simulink model "simRobotArmWith2Links"  (R2014b)
settings: Solver=ode5  StartTime=0.0  StopTime=tf  FixedStep=dt  MaxStep=dtmax  RelTol=1e-3
values from neighbouring files (symbols this model uses):
  alpha = 1    [robotArmWith2Links.m]    (also in threeLinkFTC.m; twoLinkFTC.m; twoLinkFTCwAdaptive.m)
  Ar = [0 5; -30 -30]    [robotArmWith2Links.m]    (also in threeLinkFTC.m = [0 1; -5 -5]; twoLinkFTC.m = [0 10; -40 -40]; twoLinkFTCwAdaptive.m = [0 5; -250 -250])
  Arm1 = [0 1; -wn^2 -2*ksi*wn]    [robotArmWith2Links.m]    (also in threeLinkFTC.m; twoLinkFTC.m; twoLinkFTCwAdaptive.m)
  Bfault = [0 0; 0 1]    [robotArmWith2Links.m]    (also in threeLinkFTC.m; twoLinkFTC.m; twoLinkFTCwAdaptive.m)
  Brm1 = [0 wn^2]'    [robotArmWith2Links.m]    (also in threeLinkFTC.m; twoLinkFTC.m; twoLinkFTCwAdaptive.m)
  dt = 1e-3    (= 0.001)    [robotArmWith2Links.m]
  dtFC = dt    (= 0.001)    [robotArmWith2Links.m]
  epsilon = 0.5    [robotArmWith2Links.m]    (also in threeLinkFTC.m; twoLinkFTC.m; twoLinkFTCwAdaptive.m)
  g = 9.81    [robotArmWith2Links.m]    (also in threeLinkFTC.m; twoLinkFDIbasisComparison.m; twoLinkFTC.m; twoLinkFTCwAdaptive.m)
  I1 = 8.33e-2    (= 0.0833)    [robotArmWith2Links.m]    (also in threeLinkFTC.m = 0.0833333333333; twoLinkFDIbasisComparison.m = 0.0833333333333; twoLinkFTC.m = 0.0833333333333; twoLinkFTCwAdaptive.m = 0.0833333333333)
  I2 = 8.33e-2    (= 0.0833)    [robotArmWith2Links.m]    (also in threeLinkFTC.m = 0.0833333333333; twoLinkFDIbasisComparison.m = 0.0833333333333; twoLinkFTC.m = 0.0833333333333; twoLinkFTCwAdaptive.m = 0.0833333333333)
  K1 = 2*wn*ksi    (= 87.9645943005)    [robotArmWith2Links.m]    (also in threeLinkFTC.m = 8.79645943005; twoLinkFTC.m; twoLinkFTCwAdaptive.m = 43.9822971503)
  K2 = wn^2    (= 986.960440109)    [robotArmWith2Links.m]    (also in threeLinkFTC.m = 39.4784176044; twoLinkFTC.m; twoLinkFTCwAdaptive.m)
  l1 = 1    [robotArmWith2Links.m]    (also in threeLinkFTC.m; twoLinkFDIbasisComparison.m; twoLinkFTC.m; twoLinkFTCwAdaptive.m)
  l2 = 1    [robotArmWith2Links.m]    (also in threeLinkFTC.m; twoLinkFDIbasisComparison.m; twoLinkFTC.m; twoLinkFTCwAdaptive.m)
  lc1 = l1/2    (= 0.5)    [robotArmWith2Links.m]    (also in threeLinkFTC.m; twoLinkFDIbasisComparison.m; twoLinkFTC.m; twoLinkFTCwAdaptive.m)
  lc2 = l2/2    (= 0.5)    [robotArmWith2Links.m]    (also in threeLinkFTC.m; twoLinkFDIbasisComparison.m; twoLinkFTC.m; twoLinkFTCwAdaptive.m)
  m1 = 1    [robotArmWith2Links.m]    (also in threeLinkFTC.m; twoLinkFDIbasisComparison.m; twoLinkFTC.m; twoLinkFTCwAdaptive.m)
  m2 = 1    [robotArmWith2Links.m]    (also in threeLinkFTC.m; twoLinkFDIbasisComparison.m; twoLinkFTC.m; twoLinkFTCwAdaptive.m)
  q0 = [80 20]'*pi/180    [robotArmWith2Links.m]    (also in threeLinkFTC.m = [90 0 0]'*pi/180; twoLinkFDIbasisComparison.m = [90 0]'*pi/180; twoLinkFTC.m = [90 0]'*pi/180; twoLinkFTCwAdaptive.m = [90 0]'*pi/180)
  qdot0 = [0 0]'    [robotArmWith2Links.m]    (also in threeLinkFTC.m = [0 0 0]'*pi/180; twoLinkFDIbasisComparison.m = [0 0]'*pi/180; twoLinkFTC.m = [0 0]'*pi/180; twoLinkFTCwAdaptive.m = [0 0]'*pi/180)
  r0 = [0 0]'    [robotArmWith2Links.m]    (also in threeLinkFTC.m; twoLinkFTC.m; twoLinkFTCwAdaptive.m)
  rmax = inf*[50*pi/180 inf]'    [robotArmWith2Links.m]    (also in threeLinkFTC.m; twoLinkFTC.m; twoLinkFTCwAdaptive.m)
  rmin = -rmax    [robotArmWith2Links.m]    (also in threeLinkFTC.m; twoLinkFTC.m; twoLinkFTCwAdaptive.m)
  visualFlag = 0    [robotArmWith2Links.m]    (also in twoLinkFDIbasisComparison.m; twoLinkFTC.m; twoLinkFTCwAdaptive.m)
  visualizationDataFlag = 1    [robotArmWith2Links.m]    (also in twoLinkFDIbasisComparison.m; twoLinkFTC.m; twoLinkFTCwAdaptive.m)
undefined symbols (not defined in the file or in its folder): twolinkplot
libraries: simulink x1
(part 1 of 2)
settings Model: Creator=alp.marangoz  LastModifiedBy=alpmarangoz
settings SolverCC: AutoInsertRateTranBlk=on
settings DataIOCC: SignalLoggingSaveFormat=ModelDataLogs
settings OptimizationCC: InlineParams=on  InlineInvariantSignals=on  ExpressionDepthLimit=2147483647  EfficientFloat2IntCast=on
settings DebuggingCC: UnderspecifiedInitializationDetection=Classic  MergeDetectMultiDrivingBlocksExec=none  FcnCallInpInsideContextMsg=UseLocalSettings  UniqueDataStoreMsg=error  StateNameClashWarn=warning
settings GRTTargetCC: CombineOutputUpdateFcns=off  GRTInterface=on

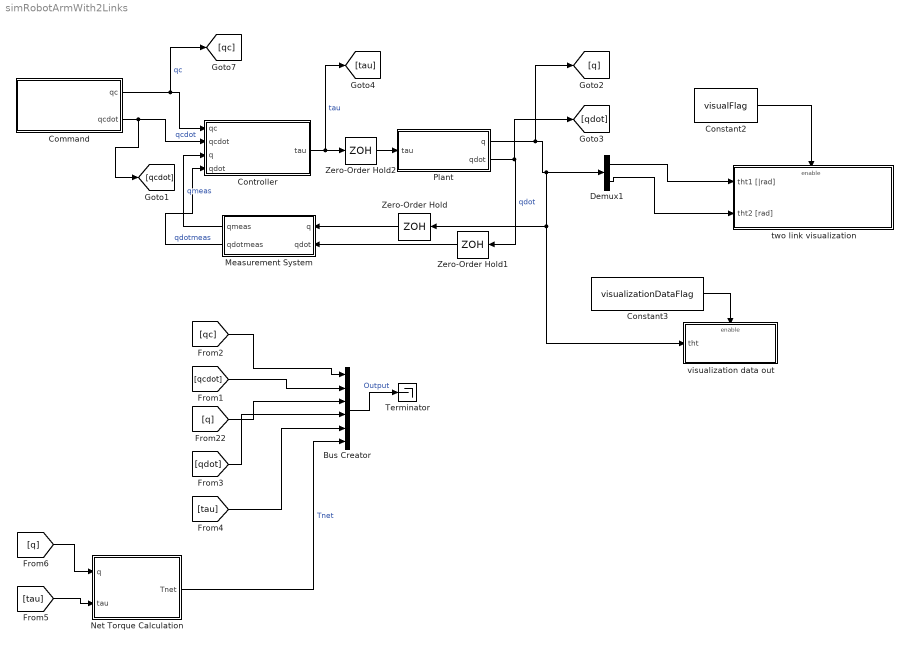
== system simRobotArmWith2Links ==
  Bus Creator : BusCreator  Inputs=6
  Command : Subsystem  TreatAsAtomicUnit=on  SystemSampleTime=dtFC
  Constant2 : Constant  Value=visualFlag
  Constant3 : Constant  Value=visualizationDataFlag
  Controller : Subsystem  TreatAsAtomicUnit=on  SystemSampleTime=dtFC
  Demux1 : Demux  Outputs=2
  Measurement System : Subsystem  TreatAsAtomicUnit=on  SystemSampleTime=dtFC
  Net Torque Calculation : Subsystem
  Plant : Subsystem  TreatAsAtomicUnit=on
  Terminator : Terminator
  Zero-Order Hold : ZeroOrderHold  SampleTime=dtFC
  Zero-Order Hold1 : ZeroOrderHold  SampleTime=dtFC
  Zero-Order Hold2 : ZeroOrderHold  SampleTime=dtFC
  two link visualization : Subsystem
  visualization data out : Subsystem  TreatAsAtomicUnit=on
  wires:
  Constant2/1 -> two link visualization/Enable
  Demux1/1 -> two link visualization/1(tht1 [|rad])
  Demux1/2 -> two link visualization/2(tht2 [rad])
  Command/1(qc) -> [qc], Controller/1(qc)  "qc"
  Command/2(qcdot) -> [qcdot], Controller/2(qcdot)  "qcdot"
  Measurement System/1(qmeas) -> Controller/3(q)  "qmeas"
  Measurement System/2(qdotmeas) -> Controller/4(qdot)  "qdotmeas"
  Constant3/1 -> visualization data out/Enable
  Controller/1(tau) -> [tau], Zero-Order Hold2/1  "tau"
  Plant/1(q) -> [q], Demux1/1, visualization data out/1(tht), Zero-Order Hold/1
  Plant/2(qdot) -> [qdot], Zero-Order Hold1/1  "qdot"
  Zero-Order Hold/1 -> Measurement System/1(q)
  Zero-Order Hold1/1 -> Measurement System/2(qdot)
  Zero-Order Hold2/1 -> Plant/1(tau)
  Bus Creator/1 -> Terminator/1  "Output"
  [qcdot] -> Bus Creator/2
  [q] -> Bus Creator/3
  [qc] -> Bus Creator/1
  [qdot] -> Bus Creator/4
  [tau] -> Bus Creator/5
  [tau] -> Net Torque Calculation/2(tau)
  [q] -> Net Torque Calculation/1(q)
  Net Torque Calculation/1(Tnet) -> Bus Creator/6  "Tnet"

== system simRobotArmWith2Links/Command ==
  From Workspace : FromWorkspace  VariableName=qcData  OutputAfterFinalValue=Setting to zero
  From Workspace1 : FromWorkspace  VariableName=qcdotData  OutputAfterFinalValue=Setting to zero
  Reshape : Reshape  OutputDimensionality=Column vector (2-D)
  Reshape1 : Reshape  OutputDimensionality=Column vector (2-D)
  qc : Outport
  qcdot : Outport  Port=2
  wires:
  From Workspace/1 -> Reshape/1  "qc"
  From Workspace1/1 -> Reshape1/1  "qcdot"
  Reshape/1 -> qc/1  "qc"
  Reshape1/1 -> qcdot/1  "qcdot"

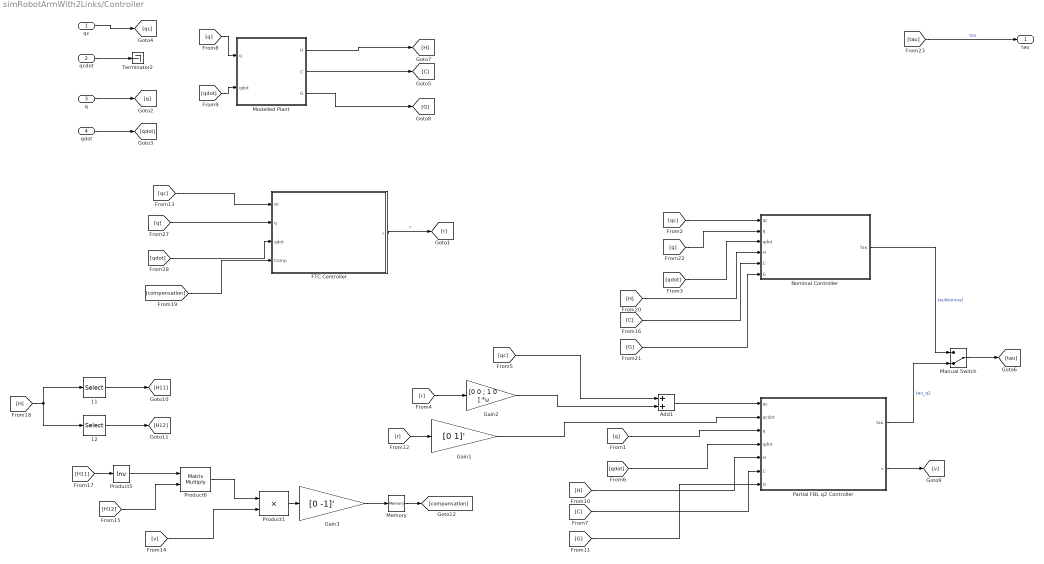
== system simRobotArmWith2Links/Controller ==
  qc : Inport
  qcdot : Inport  Port=2
  q : Inport  Port=3
  qdot : Inport  Port=4
  " FTC Controller" : Subsystem  TreatAsAtomicUnit=on
  11 : Selector  NumberOfDimensions=2  InputPortWidth=3  IndexOptions=Index vector (dialog),Index vector (dialog)  Indices=1,1  OutputSizes=1,1
  12 : Selector  NumberOfDimensions=2  InputPortWidth=3  IndexOptions=Index vector (dialog),Index vector (dialog)  Indices=1,2  OutputSizes=1,1
  Add1 : Sum
  Gain1 : Gain  Gain=[0 1]'
  Gain2 : Gain  Gain=[0 0 ; 1 0 ]  Multiplication=Matrix(K*u)
  Gain3 : Gain  Gain=[0 -1]'
  Manual Switch : ManualSwitch  CurrentSetting=0
  Memory : Memory  InheritSampleTime=on  LinearizeMemory=on  LinearizeAsDelay=on
  Modelled Plant : Subsystem  TreatAsAtomicUnit=on
  Nominal Controller : Subsystem  TreatAsAtomicUnit=on
  Partial FBL q2 Controller : Subsystem
  Product1 : Product  RndMeth=Zero
  Product5 : Product  Inputs=/  Multiplication=Matrix(*)  RndMeth=Zero
  Product6 : Product  Multiplication=Matrix(*)  RndMeth=Zero
  Terminator2 : Terminator
  tau : Outport
  wires:
  q/1 -> [q]
  qdot/1 -> [qdot]
  qc/1 -> [qc]
  qcdot/1 -> Terminator2/1
  [qc] -> " FTC Controller"/1(qc)
  [q] -> " FTC Controller"/2(q)
  [qdot] -> " FTC Controller"/3(qdot)
  " FTC Controller"/1(r) -> [r]  "r"
  [q] -> Modelled Plant/1(q)
  [qdot] -> Modelled Plant/2(qdot)
  Modelled Plant/1(H) -> [H]
  Modelled Plant/2(C) -> [C]
  Modelled Plant/3(G) -> [G]
  [q] -> Nominal Controller/2(q)
  [H] -> Nominal Controller/4(H)
  [C] -> Nominal Controller/5(C)
  [G] -> Nominal Controller/6(G)
  [qdot] -> Nominal Controller/3(qdot)
  [tau] -> tau/1  "tau"
  [qc] -> Nominal Controller/1(qc)
  Manual Switch/1 -> [tau]
  Nominal Controller/1(tau) -> Manual Switch/1  "tauNominal"
  Partial FBL q2 Controller/1(tau) -> Manual Switch/2  "tau_q2"
  Gain2/1 -> Add1/2
  [qc] -> Add1/1
  [r] -> Gain2/1
  Add1/1 -> Partial FBL q2 Controller/1(qc)
  [q] -> Partial FBL q2 Controller/3(q)
  [qdot] -> Partial FBL q2 Controller/4(qdot)
  [H] -> Partial FBL q2 Controller/5(H)
  [C] -> Partial FBL q2 Controller/6(C)
  [G] -> Partial FBL q2 Controller/7(G)
  Partial FBL q2 Controller/2(v) -> [v]
  [r] -> Gain1/1
  Gain1/1 -> Partial FBL q2 Controller/2(qcdot)
  [H11] -> Product5/1
  [H] -> 12/1, 11/1
  11/1 -> [H11]
  12/1 -> [H12]
  Product5/1 -> Product6/1
  [H12] -> Product6/2
  Product1/1 -> Gain3/1
  Product6/1 -> Product1/1
  [v] -> Product1/2
  Gain3/1 -> Memory/1
  Memory/1 -> [compensation]
  [compensation] -> " FTC Controller"/4(Comp)

== system simRobotArmWith2Links/Measurement System ==
  q : Inport
  qdot : Inport  Port=2
  Constant : Constant  Value=2*pi
  Math Function : Math  Operator=rem  SaturateOnIntegerOverflow=on
  Memory : Memory  X0=q0  InheritSampleTime=on  LinearizeMemory=on  LinearizeAsDelay=on
  Memory1 : Memory  X0=qdot0  InheritSampleTime=on  LinearizeMemory=on  LinearizeAsDelay=on
  qmeas : Outport
  qdotmeas : Outport  Port=2
  wires:
  q/1 -> [q]  "q"
  qdot/1 -> [qdot]  "qdot"
  [qdotmeas] -> qdotmeas/1  "qdotmeas"
  [qmeas] -> qmeas/1  "qmeas"
  [qdot] -> Memory1/1
  Memory1/1 -> [qdotmeas]
  Constant/1 -> Math Function/2
  [q] -> Memory/1  "q"
  Memory/1 -> Math Function/1
  Math Function/1 -> [qmeas]  "qrem"

== system simRobotArmWith2Links/Net Torque Calculation ==
  q : Inport
  tau : Inport  Port=2
  Add : Sum  Inputs=+++
  Add1 : Sum
  Demux1 : Demux  Outputs=2
  Demux2 : Demux  Outputs=2
  Gain : Gain  Gain=(m1*lc1+m2*l1)*g
  Gain1 : Gain  Gain=m2*g*lc2
  Gain3 : Gain  Gain=m2*g*lc2
  Mux : Mux  Inputs=2
  Reshape : Reshape  OutputDimensionality=Column vector (2-D)
  Sum of Elements : Sum  Inputs=+
  Terminator1 : Terminator
  Terminator5 : Terminator
  Trigonometric Function1 : Trigonometry  Operator=cos
  Trigonometric Function3 : Trigonometry  Operator=cos
  Tnet : Outport
  wires:
  Demux2/1 -> [c1]
  Demux2/2 -> Terminator5/1
  Trigonometric Function1/1 -> Demux2/1
  Sum of Elements/1 -> Trigonometric Function3/1
  Trigonometric Function3/1 -> [c12]
  q/1 -> Sum of Elements/1, Trigonometric Function1/1
  [c1] -> Gain/1
  Gain/1 -> Add/1  "term1"
  [c12] -> Gain1/1
  Gain1/1 -> Add/2  "term2"
  [c12] -> Gain3/1
  Gain3/1 -> Add1/2
  [tau2] -> Add/3  "term3"
  [tau2] -> Add1/1
  Demux1/1 -> Terminator1/1
  Demux1/2 -> [tau2]
  tau/1 -> Demux1/1
  Mux/1 -> Reshape/1
  Add/1 -> Mux/1
  Add1/1 -> Mux/2
  Reshape/1 -> Tnet/1

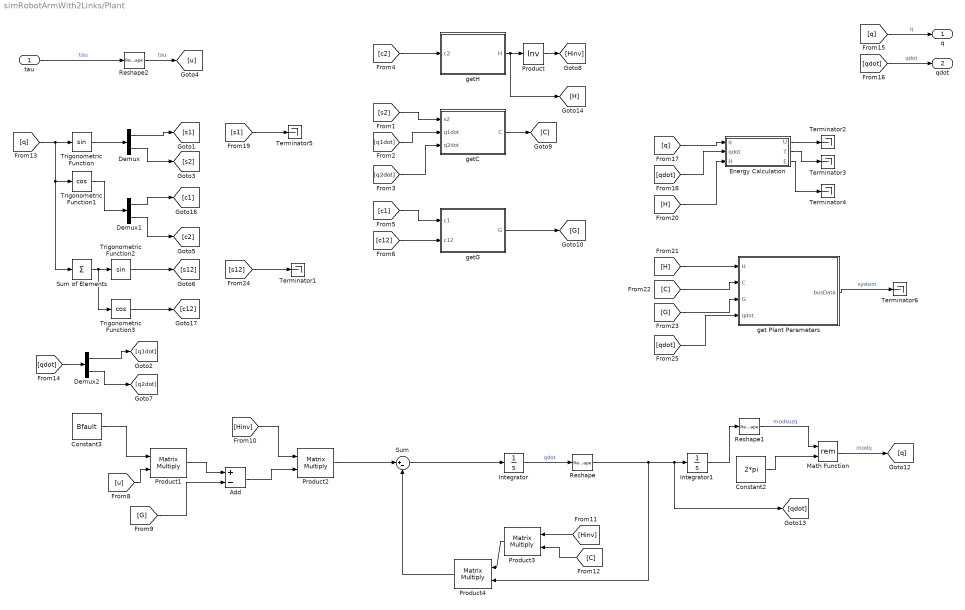
== system simRobotArmWith2Links/Plant ==
  tau : Inport
  Add : Sum  Inputs=+-
  Constant2 : Constant  Value=2*pi
  Constant3 : Constant  Value=Bfault  VectorParams1D=off
  Demux : Demux  Outputs=2
  Demux1 : Demux  Outputs=2
  Demux2 : Demux  Outputs=2
  Energy Calculation : Subsystem
  Integrator : Integrator  InitialCondition=qdot0  UpperSaturationLimit=10000*pi/180  LowerSaturationLimit=-10000*pi/180
  Integrator1 : Integrator  InitialCondition=q0
  Math Function : Math  Operator=rem  SaturateOnIntegerOverflow=on
  Product : Product  Inputs=/  Multiplication=Matrix(*)  RndMeth=Zero
  Product{1..4} (4 alike) : Product  Multiplication=Matrix(*)  RndMeth=Zero
  Reshape : Reshape  OutputDimensionality=Column vector (2-D)
  Reshape1 : Reshape  OutputDimensionality=Column vector (2-D)
  Reshape2 : Reshape  OutputDimensionality=Column vector (2-D)
  Sum : Sum  Inputs=|+-
  Sum of Elements : Sum  Inputs=+
  Terminator{1..6} (6 alike) : Terminator
  Trigonometric Function : Trigonometry
  Trigonometric Function1 : Trigonometry  Operator=cos
  Trigonometric Function2 : Trigonometry
  Trigonometric Function3 : Trigonometry  Operator=cos
  get Plant Parameters : Subsystem
  getC : Subsystem
  getG : Subsystem
  getH : Subsystem
  q : Outport
  qdot : Outport  Port=2
  wires:
  [q] -> Trigonometric Function/1, Trigonometric Function1/1, Sum of Elements/1
  Trigonometric Function/1 -> Demux/1
  Demux/1 -> [s1]
  Demux/2 -> [s2]
  Demux1/1 -> [c1]
  Demux1/2 -> [c2]
  Trigonometric Function1/1 -> Demux1/1
  [c2] -> getH/1(c2)
  Sum of Elements/1 -> Trigonometric Function2/1, Trigonometric Function3/1
  Trigonometric Function2/1 -> [s12]
  [qdot] -> Demux2/1
  Demux2/1 -> [q1dot]
  Demux2/2 -> [q2dot]
  [s2] -> getC/1(s2)
  [q1dot] -> getC/2(q1dot)
  [q2dot] -> getC/3(q2dot)
  getH/1(H) -> Product/1, [H]
  getC/1(C) -> [C]
  [c1] -> getG/1(c1)
  [c12] -> getG/2(c12)
  getG/1(G) -> [G]
  Product/1 -> [Hinv]
  [G] -> Add/2
  [Hinv] -> Product2/1
  Add/1 -> Product2/2
  Product2/1 -> Sum/1
  [Hinv] -> Product3/1
  [C] -> Product3/2
  Product3/1 -> Product4/1
  Product4/1 -> Sum/2
  Sum/1 -> Integrator/1
  Integrator/1 -> Reshape/1  "qdot"
  Integrator1/1 -> Reshape1/1
  [q] -> q/1  "q"
  [qdot] -> qdot/1  "qdot"
  Reshape/1 -> Product4/2, [qdot], Integrator1/1
  Reshape2/1 -> [u]  "tau"
  tau/1 -> Reshape2/1  "tau"
  Trigonometric Function3/1 -> [c12]
  [s12] -> Terminator1/1
  [q] -> Energy Calculation/1(q)
  [qdot] -> Energy Calculation/2(qdot)
  Energy Calculation/1(U) -> Terminator2/1
  Energy Calculation/2(T) -> Terminator3/1
  Energy Calculation/3(E) -> Terminator4/1
  [s1] -> Terminator5/1
  [H] -> Energy Calculation/3(H)
  Reshape1/1 -> Math Function/1  "modsuzq"
  Constant2/1 -> Math Function/2
  Math Function/1 -> [q]  "modq"
  get Plant Parameters/1(busData) -> Terminator6/1  "system"
  [C] -> get Plant Parameters/2(C)
  [H] -> get Plant Parameters/1(H)
  [G] -> get Plant Parameters/3(G)
  [qdot] -> get Plant Parameters/4(qdot)
  [u] -> Product1/2
  Product1/1 -> Add/1
  Constant3/1 -> Product1/1

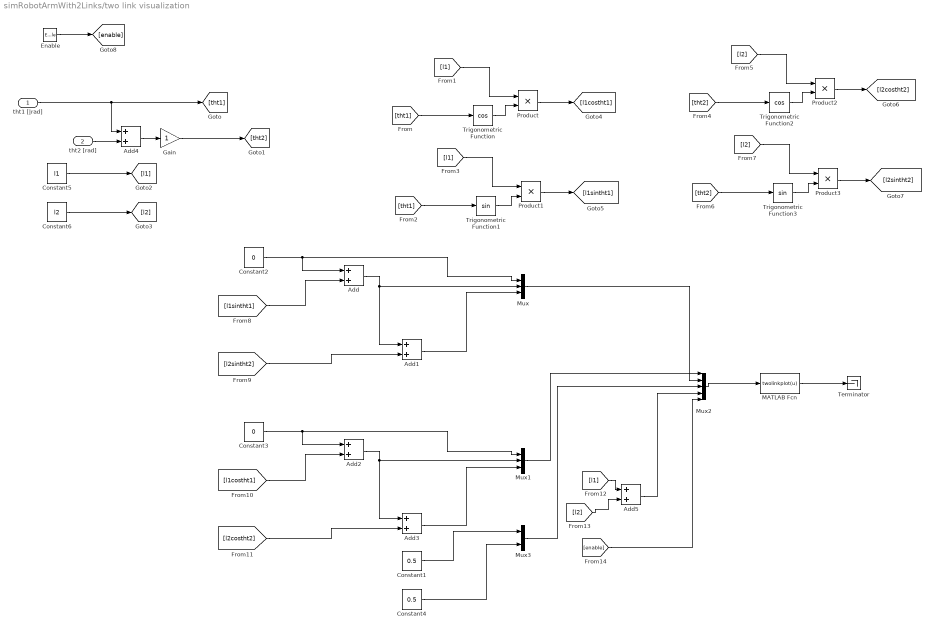
== system simRobotArmWith2Links/two link visualization ==
  tht1 [|rad] : Inport
  tht2 [rad] : Inport  Port=2
  Enable : EnablePort  PropagateVarSize=During execution  ShowOutputPort=on
  Add{,1..5} (6 alike) : Sum
  Constant1 : Constant  Value=0.5
  Constant2 : Constant  Value=0
  Constant3 : Constant  Value=0
  Constant4 : Constant  Value=0.5
  Constant5 : Constant  Value=l1  VectorParams1D=off
  Constant6 : Constant  Value=l2  VectorParams1D=off
  Gain : Gain
  MATLAB Fcn : MATLABFcn  MATLABFcn=twolinkplot(u)
  Mux : Mux  Inputs=3
  Mux1 : Mux  Inputs=3
  Mux2 : Mux  Inputs=5
  Mux3 : Mux  Inputs=2
  Product{,1..3} (4 alike) : Product  RndMeth=Zero
  Terminator : Terminator
  Trigonometric Function : Trigonometry  Operator=cos
  Trigonometric Function1 : Trigonometry
  Trigonometric Function2 : Trigonometry  Operator=cos
  Trigonometric Function3 : Trigonometry
  wires:
  [tht1] -> Trigonometric Function/1
  Constant5/1 -> [l1]
  Constant6/1 -> [l2]
  [l1] -> Product/1
  Trigonometric Function/1 -> Product/2
  Product/1 -> [l1costht1]
  [tht1] -> Trigonometric Function1/1
  [l1] -> Product1/1
  Trigonometric Function1/1 -> Product1/2
  Product1/1 -> [l1sintht1]
  [tht2] -> Trigonometric Function2/1
  [l2] -> Product2/1
  Trigonometric Function2/1 -> Product2/2
  Product2/1 -> [l2costht2]
  [tht2] -> Trigonometric Function3/1
  [l2] -> Product3/1
  Trigonometric Function3/1 -> Product3/2
  Product3/1 -> [l2sintht2]
  Constant2/1 -> Add/1, Mux/1
  [l1sintht1] -> Add/2
  Add/1 -> Add1/1, Mux/2
  [l2sintht2] -> Add1/2
  Add1/1 -> Mux/3
  Constant3/1 -> Mux1/1, Add2/1
  [l1costht1] -> Add2/2
  Add2/1 -> Mux1/2, Add3/1
  [l2costht2] -> Add3/2
  Add3/1 -> Mux1/3
  Mux2/1 -> MATLAB Fcn/1
  MATLAB Fcn/1 -> Terminator/1
  tht2 [rad]/1 -> Add4/2
  Gain/1 -> [tht2]
  Add4/1 -> Gain/1
  [l1] -> Add5/1
  [l2] -> Add5/2
  Enable/1 -> [enable]
  Constant1/1 -> Mux3/1
  Constant4/1 -> Mux3/2
  Mux3/1 -> Mux2/3
  Add5/1 -> Mux2/4
  [enable] -> Mux2/5
  tht1 [|rad]/1 -> Add4/1, [tht1]
  Mux1/1 -> Mux2/1
  Mux/1 -> Mux2/2

== system simRobotArmWith2Links/visualization data out ==
  tht : Inport
  Enable : EnablePort  PropagateVarSize=During execution
  To Workspace : ToWorkspace  VariableName=thetaForVisualization  SaveFormat=Structure With Time  SampleTime=-1
  wires:
  tht/1 -> To Workspace/1

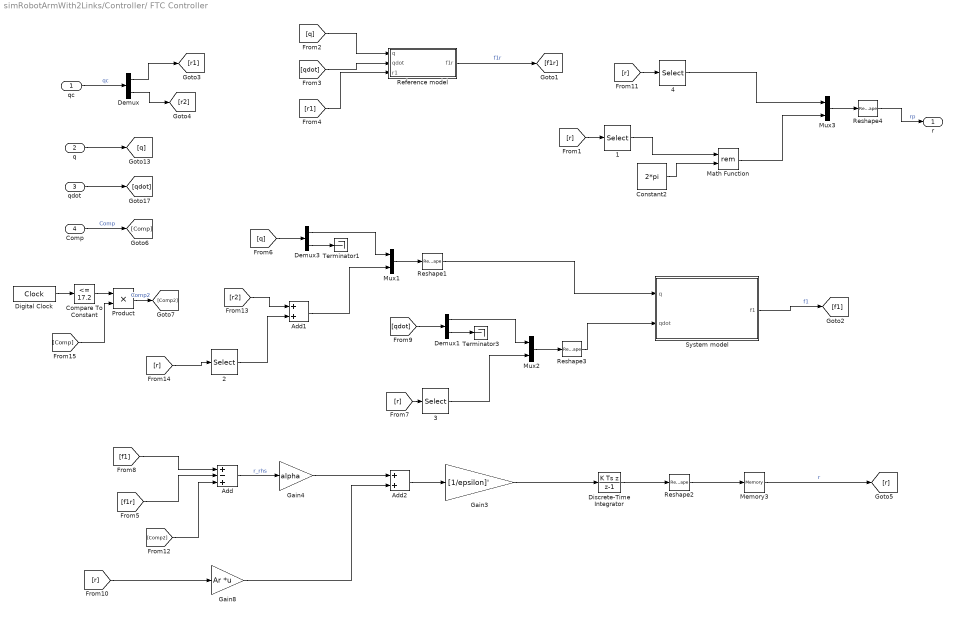
== system simRobotArmWith2Links/Controller/ FTC Controller ==
  qc : Inport
  q : Inport  Port=2
  qdot : Inport  Port=3
  Comp : Inport  Port=4
  1 : Selector  NumberOfDimensions=2  InputPortWidth=3  IndexOptions=Index vector (dialog),Index vector (dialog)  Indices=1,1  OutputSizes=1,1
  2 : Selector  NumberOfDimensions=2  InputPortWidth=3  IndexOptions=Index vector (dialog),Index vector (dialog)  Indices=1,1  OutputSizes=1,1
  3 : Selector  NumberOfDimensions=2  InputPortWidth=3  IndexOptions=Index vector (dialog),Index vector (dialog)  Indices=2,1  OutputSizes=1,1
  4 : Selector  NumberOfDimensions=2  InputPortWidth=3  IndexOptions=Index vector (dialog),Index vector (dialog)  Indices=2,1  OutputSizes=1,1
  Add : Sum  Inputs=+-+
  Add1 : Sum
  Add2 : Sum
  Compare To Constant : simulink/Logic and Bit Operations/Compare To Constant  relop=<=  const=17.2  OutDataTypeStr=uint8
  Constant2 : Constant  Value=2*pi
  Demux : Demux  Outputs=2
  Demux1 : Demux  Outputs=2
  Demux3 : Demux  Outputs=2
  Digital Clock : DigitalClock  SampleTime=dt
  Discrete-Time Integrator : DiscreteIntegrator  IntegratorMethod=Integration: Backward Euler  InitialCondition=r0  InitialConditionSetting=State (most efficient)  SampleTime=-1  LimitOutput=on  UpperSaturationLimit=rmax  LowerSaturationLimit=rmin
  Gain3 : Gain  Gain=[1/epsilon]'
  Gain4 : Gain  Gain=alpha
  Gain8 : Gain  Gain=Ar  Multiplication=Matrix(K*u)
  Math Function : Math  Operator=rem  SaturateOnIntegerOverflow=on
  Memory3 : Memory  X0=r0  InheritSampleTime=on  LinearizeMemory=on  LinearizeAsDelay=on
  Mux1 : Mux  Inputs=2
  Mux2 : Mux  Inputs=2
  Mux3 : Mux  Inputs=2
  Product : Product
  Reference model : Subsystem  TreatAsAtomicUnit=on
  Reshape{1..4} (4 alike) : Reshape  OutputDimensionality=Column vector (2-D)
  System model : Subsystem  TreatAsAtomicUnit=on
  Terminator1 : Terminator
  Terminator3 : Terminator
  r : Outport
  wires:
  qc/1 -> Demux/1  "qc"
  Add/1 -> Gain4/1  "r_rhs"
  [f1] -> Add/1
  [f1r] -> Add/2
  Gain4/1 -> Add2/1
  Add2/1 -> Gain3/1
  q/1 -> [q]
  qdot/1 -> [qdot]
  [qdot] -> Reference model/2(qdot)
  [q] -> Reference model/1(q)
  [r1] -> Reference model/3(r1)
  Reference model/1(f1r) -> [f1r]  "f1r"
  System model/1(f1) -> [f1]  "f1"
  Gain8/1 -> Add2/2
  Reshape3/1 -> System model/2(qdot)
  Demux3/1 -> Mux1/1
  Mux1/1 -> Reshape1/1
  Reshape1/1 -> System model/1(q)
  [q] -> Demux3/1
  Demux3/2 -> Terminator1/1
  [r2] -> Add1/1
  Add1/1 -> Mux1/2
  Memory3/1 -> [r]  "r"
  Constant2/1 -> Math Function/2
  [r] -> 1/1
  Gain3/1 -> Discrete-Time Integrator/1
  Discrete-Time Integrator/1 -> Reshape2/1
  Reshape2/1 -> Memory3/1
  Demux/1 -> [r1]
  Demux/2 -> [r2]
  [r] -> 2/1
  2/1 -> Add1/2
  Demux1/1 -> Mux2/1
  Mux2/1 -> Reshape3/1
  [qdot] -> Demux1/1
  Demux1/2 -> Terminator3/1
  3/1 -> Mux2/2
  [r] -> 3/1
  1/1 -> Math Function/1
  [r] -> Gain8/1
  4/1 -> Mux3/1
  Mux3/1 -> Reshape4/1
  Math Function/1 -> Mux3/2
  Reshape4/1 -> r/1  "rp"
  [r] -> 4/1
  Comp/1 -> [Comp]  "Comp"
  [Comp2] -> Add/3
  Digital Clock/1 -> Compare To Constant/1
  Compare To Constant/1 -> Product/1
  [Comp] -> Product/2
  Product/1 -> [Comp2]  "Comp2"

== system simRobotArmWith2Links/Controller/Modelled Plant ==
  q : Inport
  qdot : Inport  Port=2
  Demux : Demux  Outputs=2
  Demux1 : Demux  Outputs=2
  Demux2 : Demux  Outputs=2
  Sum of Elements : Sum  Inputs=+
  Terminator4 : Terminator
  Terminator5 : Terminator
  Terminator6 : Terminator
  Trigonometric Function : Trigonometry
  Trigonometric Function1 : Trigonometry  Operator=cos
  Trigonometric Function2 : Trigonometry
  Trigonometric Function3 : Trigonometry  Operator=cos
  get Plant Parameters : Subsystem
  getC : Subsystem
  getG : Subsystem
  getH : Subsystem
  H : Outport
  C : Outport  Port=2
  G : Outport  Port=3
  wires:
  [c2] -> getH/1(c2)
  [s2] -> getC/1(s2)
  [q1dot] -> getC/2(q1dot)
  [q2dot] -> getC/3(q2dot)
  getH/1(H) -> [H]
  getC/1(C) -> [C]
  [c1] -> getG/1(c1)
  [c12] -> getG/2(c12)
  getG/1(G) -> [G]
  q/1 -> Trigonometric Function/1, Trigonometric Function1/1, Sum of Elements/1
  Trigonometric Function/1 -> Demux/1
  Demux/1 -> Terminator4/1
  Demux/2 -> [s2]
  Demux1/1 -> [c1]
  Demux1/2 -> [c2]
  Trigonometric Function1/1 -> Demux1/1
  Sum of Elements/1 -> Trigonometric Function2/1, Trigonometric Function3/1
  Trigonometric Function2/1 -> Terminator5/1
  qdot/1 -> Demux2/1, [qdot]
  Demux2/1 -> [q1dot]
  Demux2/2 -> [q2dot]
  Trigonometric Function3/1 -> [c12]
  [H] -> H/1
  [C] -> C/1
  [G] -> G/1
  get Plant Parameters/1(busData) -> Terminator6/1  "modeled system"
  [C] -> get Plant Parameters/2(C)
  [H] -> get Plant Parameters/1(H)
  [G] -> get Plant Parameters/3(G)
  [qdot] -> get Plant Parameters/4(qdot)

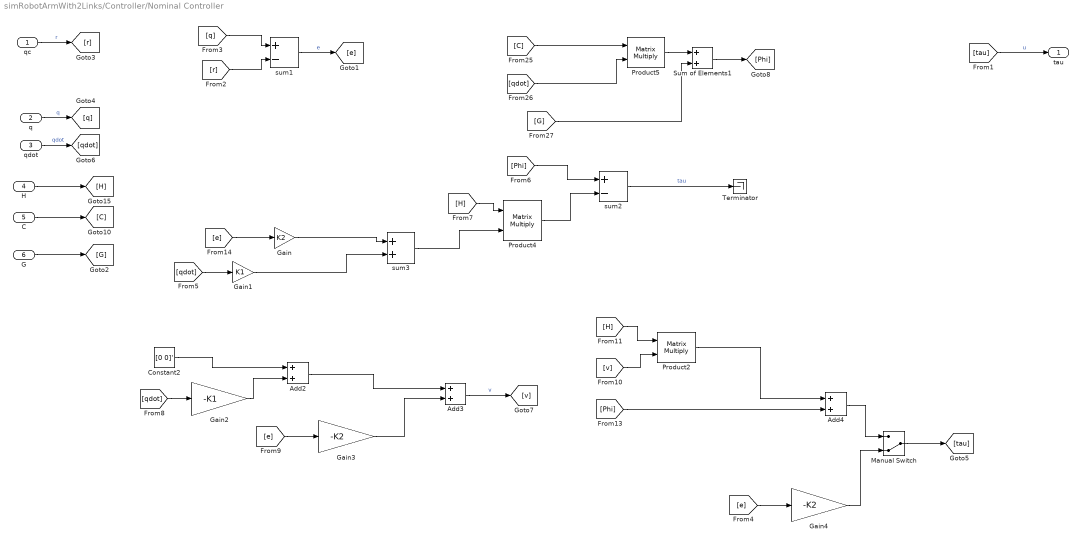
== system simRobotArmWith2Links/Controller/Nominal Controller ==
  qc : Inport
  q : Inport  Port=2
  qdot : Inport  Port=3
  H : Inport  Port=4
  C : Inport  Port=5
  G : Inport  Port=6
  Add2 : Sum
  Add3 : Sum
  Add4 : Sum
  Constant2 : Constant  Value=[0 0]'
  Gain : Gain  Gain=K2
  Gain1 : Gain  Gain=K1
  Gain2 : Gain  Gain=-K1
  Gain3 : Gain  Gain=-K2
  Gain4 : Gain  Gain=-K2
  Manual Switch : ManualSwitch  CurrentSetting=0
  Product2 : Product  Multiplication=Matrix(*)  RndMeth=Zero
  Product4 : Product  Multiplication=Matrix(*)  RndMeth=Zero
  Product5 : Product  Multiplication=Matrix(*)  RndMeth=Zero
  Sum of Elements1 : Sum
  Terminator : Terminator
  sum1 : Sum  Inputs=+-
  sum2 : Sum  Inputs=+-
  sum3 : Sum
  tau : Outport
  wires:
  G/1 -> [G]
  H/1 -> [H]
  C/1 -> [C]
  [tau] -> tau/1  "u"
  Gain1/1 -> sum3/2
  Gain/1 -> sum3/1
  qc/1 -> [r]  "r"
  sum1/1 -> [e]  "e"
  [r] -> sum1/2
  [q] -> sum1/1
  q/1 -> [q]  "q"
  qdot/1 -> [qdot]  "qdot"
  [C] -> Product5/1
  [qdot] -> Product5/2
  Product5/1 -> Sum of Elements1/1
  [G] -> Sum of Elements1/2
  Sum of Elements1/1 -> [Phi]
  sum2/1 -> Terminator/1  "tau"
  [H] -> Product4/1
  [Phi] -> sum2/1
  Product4/1 -> sum2/2
  [e] -> Gain/1
  [qdot] -> Gain1/1
  sum3/1 -> Product4/2
  [v] -> Product2/2
  Product2/1 -> Add4/1
  [Phi] -> Add4/2
  [H] -> Product2/1
  [qdot] -> Gain2/1
  Constant2/1 -> Add2/1
  Gain2/1 -> Add2/2
  [e] -> Gain3/1
  Add2/1 -> Add3/1
  Gain3/1 -> Add3/2
  Add3/1 -> [v]  "v"
  [e] -> Gain4/1
  Manual Switch/1 -> [tau]
  Add4/1 -> Manual Switch/1
  Gain4/1 -> Manual Switch/2

== system simRobotArmWith2Links/Controller/Partial FBL q2 Controller ==
  qc : Inport
  qcdot : Inport  Port=2
  q : Inport  Port=3
  qdot : Inport  Port=4
  H : Inport  Port=5
  C : Inport  Port=6
  G : Inport  Port=7
  Collocated q2 Controller : Subsystem  TreatAsAtomicUnit=on
  Constant : Constant  Value=0
  Demux{,1..3} (4 alike) : Demux  Outputs=2
  Mux : Mux  Inputs=2
  Reshape2 : Reshape  OutputDimensionality=Column vector (2-D)
  Terminator{1..4} (4 alike) : Terminator
  Torque calculation : Subsystem  TreatAsAtomicUnit=on
  tau : Outport
  v : Outport  Port=2
  wires:
  [q] -> Collocated q2 Controller/3(q)
  Collocated q2 Controller/1(v) -> [v]  "v"
  C/1 -> [C]
  H/1 -> [H]
  qc/1 -> Demux/1
  Demux/1 -> Terminator2/1
  Demux/2 -> [r]
  G/1 -> [G]
  Torque calculation/1(tau) -> [tau]
  [v] -> Torque calculation/1(v)
  [H] -> Torque calculation/2(H)
  [C] -> Torque calculation/3(C)
  [G] -> Torque calculation/4(G)
  [r] -> Collocated q2 Controller/1(r)
  q/1 -> Demux1/1
  Demux1/1 -> Terminator1/1
  Demux1/2 -> [q]
  Reshape2/1 -> tau/1  "tau"
  Constant/1 -> Mux/1
  [tau] -> Mux/2
  Mux/1 -> Reshape2/1
  [qdot] -> Torque calculation/5(qdot)
  qdot/1 -> [qdot]
  [qdot] -> Demux2/1
  Demux2/2 -> Collocated q2 Controller/4(qdot)
  Demux2/1 -> Terminator3/1
  [v] -> v/1
  qcdot/1 -> Demux3/1
  Demux3/1 -> Terminator4/1
  Demux3/2 -> [rdot]
  [rdot] -> Collocated q2 Controller/2(rdot)

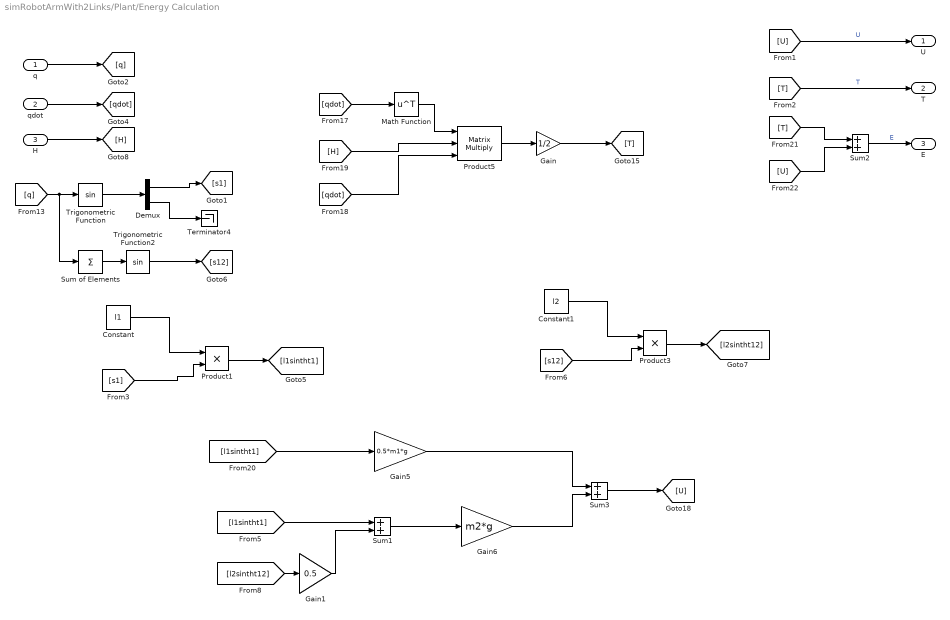
== system simRobotArmWith2Links/Plant/Energy Calculation ==
  q : Inport
  qdot : Inport  Port=2
  H : Inport  Port=3
  Constant : Constant  Value=l1  VectorParams1D=off
  Constant1 : Constant  Value=l2  VectorParams1D=off
  Demux : Demux  Outputs=2
  Gain : Gain  Gain=1/2
  Gain1 : Gain  Gain=0.5
  Gain5 : Gain  Gain=0.5*m1*g
  Gain6 : Gain  Gain=m2*g
  Math Function : Math  Operator=transpose  SaturateOnIntegerOverflow=on
  Product1 : Product  RndMeth=Zero
  Product3 : Product  RndMeth=Zero
  Product5 : Product  Inputs=3  Multiplication=Matrix(*)  RndMeth=Zero
  Sum of Elements : Sum  Inputs=+
  Sum1 : Sum
  Sum2 : Sum
  Sum3 : Sum
  Terminator4 : Terminator
  Trigonometric Function : Trigonometry
  Trigonometric Function2 : Trigonometry
  U : Outport
  T : Outport  Port=2
  E : Outport  Port=3
  wires:
  [q] -> Trigonometric Function/1, Sum of Elements/1
  Trigonometric Function/1 -> Demux/1
  Demux/1 -> [s1]
  Demux/2 -> Terminator4/1
  Sum of Elements/1 -> Trigonometric Function2/1
  Trigonometric Function2/1 -> [s12]
  [qdot] -> Math Function/1
  Math Function/1 -> Product5/1
  [H] -> Product5/2
  [qdot] -> Product5/3
  Product5/1 -> Gain/1
  [l1sintht1] -> Gain5/1
  Gain/1 -> [T]
  [l1sintht1] -> Sum1/1
  [l2sintht12] -> Gain1/1
  Gain5/1 -> Sum3/1
  Gain6/1 -> Sum3/2
  [T] -> Sum2/1
  [U] -> Sum2/2
  q/1 -> [q]
  qdot/1 -> [qdot]
  Sum2/1 -> E/1  "E"
  [U] -> U/1  "U"
  [T] -> T/1  "T"
  Constant/1 -> Product1/1
  [s1] -> Product1/2
  Product1/1 -> [l1sintht1]
  Constant1/1 -> Product3/1
  [s12] -> Product3/2
  Product3/1 -> [l2sintht12]
  Gain1/1 -> Sum1/2
  Sum1/1 -> Gain6/1
  Sum3/1 -> [U]
  H/1 -> [H]

== system simRobotArmWith2Links/Plant/get Plant Parameters ==
  H : Inport
  C : Inport  Port=2
  G : Inport  Port=3
  qdot : Inport  Port=4
  {1,5,7,11} (4 alike) : Selector  NumberOfDimensions=2  InputPortWidth=3  IndexOptions=Index vector (dialog),Index vector (dialog)  Indices=1,1  OutputSizes=1,1
  12 : Selector  NumberOfDimensions=2  InputPortWidth=3  IndexOptions=Index vector (dialog),Index vector (dialog)  Indices=1,2  OutputSizes=1,1
  2 : Selector  NumberOfDimensions=2  InputPortWidth=3  IndexOptions=Index vector (dialog),Index vector (dialog)  Indices=1,2  OutputSizes=1,1
  {3,6,8,21} (4 alike) : Selector  NumberOfDimensions=2  InputPortWidth=3  IndexOptions=Index vector (dialog),Index vector (dialog)  Indices=2,1  OutputSizes=1,1
  22 : Selector  NumberOfDimensions=2  InputPortWidth=3  IndexOptions=Index vector (dialog),Index vector (dialog)  Indices=2,2  OutputSizes=1,1
  4 : Selector  NumberOfDimensions=2  InputPortWidth=3  IndexOptions=Index vector (dialog),Index vector (dialog)  Indices=2,2  OutputSizes=1,1
  Bus Creator : BusCreator  Inputs=15
  Product5 : Product  Multiplication=Matrix(*)  RndMeth=Zero
  Sum of Elements1 : Sum
  busData : Outport
  wires:
  2/1 -> Bus Creator/9  "C12"
  21/1 -> Bus Creator/6  "H21"
  22/1 -> Bus Creator/7  "H22"
  4/1 -> Bus Creator/11  "C22"
  6/1 -> Bus Creator/13  "G_2"
  1/1 -> Bus Creator/8  "C11"
  5/1 -> Bus Creator/12  "G_1"
  12/1 -> Bus Creator/5  "H12"
  3/1 -> Bus Creator/10  "C21"
  11/1 -> Bus Creator/4  "H11"
  [H] -> 11/1, 12/1, 21/1, 22/1
  [C] -> 1/1, 2/1, 4/1, 3/1
  [G] -> 6/1, 5/1
  [C] -> Product5/1
  [qdot] -> Product5/2
  Product5/1 -> Sum of Elements1/1
  [G] -> Sum of Elements1/2
  Sum of Elements1/1 -> 7/1, 8/1
  7/1 -> Bus Creator/14  "phi1"
  8/1 -> Bus Creator/15  "phi2"
  [G] -> Bus Creator/3
  Bus Creator/1 -> busData/1
  [C] -> Bus Creator/2
  [H] -> Bus Creator/1
  H/1 -> [H]  "H"
  C/1 -> [C]  "C"
  G/1 -> [G]  "G"
  qdot/1 -> [qdot]

== system simRobotArmWith2Links/Plant/getC ==
  s2 : Inport
  q1dot : Inport  Port=2
  q2dot : Inport  Port=3
  C calculation 1 : Subsystem
  C calculation 2 : Subsystem
  Gain2 : Gain  Gain=m2*l1*lc2
  Terminator : Terminator
  C : Outport
  wires:
  s2/1 -> [s2]
  q1dot/1 -> [q1dot]
  q2dot/1 -> [q2dot]
  [s2] -> Gain2/1
  Gain2/1 -> [h]
  [q1dot] -> C calculation 1/1(q1dot)
  [q2dot] -> C calculation 1/2(q2dot)
  [h] -> C calculation 1/3(h)
  [q1dot] -> C calculation 2/1(q1dot)
  [q2dot] -> C calculation 2/2(q2dot)
  [h] -> C calculation 2/3(h)
  [C] -> C/1
  C calculation 2/1(C) -> [C]
  C calculation 1/1(C) -> Terminator/1

== system simRobotArmWith2Links/Plant/getG ==
  c1 : Inport
  c12 : Inport  Port=2
  Add : Sum
  Gain : Gain  Gain=(m1*lc1+m2*l1)*g
  Gain1 : Gain  Gain=m2*g*lc2
  Gain2 : Gain
  Gain4 : Gain  Gain=lc2*m2*g
  Matrix Concatenate2 : Concatenate  Mode=Multidimensional array
  G : Outport
  wires:
  [c12] -> Gain4/1
  Gain4/1 -> [G21]
  c12/1 -> [c12]
  c1/1 -> [c1]
  Matrix Concatenate2/1 -> Gain2/1
  [G11] -> Matrix Concatenate2/1
  [G21] -> Matrix Concatenate2/2
  [c1] -> Gain/1
  Gain/1 -> Add/1
  [c12] -> Gain1/1
  Gain1/1 -> Add/2
  Add/1 -> [G11]
  Gain2/1 -> G/1

== system simRobotArmWith2Links/Plant/getH ==
  c2 : Inport
  Constant1 : Constant  Value=I1 + I2 + m1*lc1^2 + m2*(l1^2+lc2^2)  VectorParams1D=off
  Constant2 : Constant  Value=I2+m2*lc2^2  VectorParams1D=off
  Constant3 : Constant  Value=I2+m2*lc2^2  VectorParams1D=off
  Gain : Gain  Gain=m2*2*l1*lc2
  Gain1 : Gain  Gain=m2*l1*lc2
  Matrix Concatenate : Concatenate  Mode=Multidimensional array  ConcatenateDimension=2
  Matrix Concatenate1 : Concatenate  Mode=Multidimensional array  ConcatenateDimension=2
  Matrix Concatenate2 : Concatenate  Mode=Multidimensional array
  Sum : Sum
  Sum1 : Sum
  H : Outport
  wires:
  [H11] -> Matrix Concatenate/1
  [H12] -> Matrix Concatenate/2
  Matrix Concatenate/1 -> Matrix Concatenate2/1
  Matrix Concatenate1/1 -> Matrix Concatenate2/2
  [H21] -> Matrix Concatenate1/1
  [H22] -> Matrix Concatenate1/2
  Matrix Concatenate2/1 -> H/1
  c2/1 -> [c2]
  [c2] -> Gain/1
  Gain/1 -> Sum/1
  Constant1/1 -> Sum/2
  Sum/1 -> [H11]
  [c2] -> Gain1/1
  Gain1/1 -> Sum1/1
  Constant2/1 -> Sum1/2
  Sum1/1 -> [H12], [H21]
  Constant3/1 -> [H22]

== system simRobotArmWith2Links/Controller/ FTC Controller/Reference model ==
  q : Inport
  qdot : Inport  Port=2
  r1 : Inport  Port=3
  Add : Sum
  Constant : Constant  Value=Arm1  VectorParams1D=off
  Constant1 : Constant  Value=Brm1  VectorParams1D=off
  Demux2 : Demux  Outputs=2
  Demux3 : Demux  Outputs=2
  Mux : Mux  Inputs=2
  Product1 : Product  Multiplication=Matrix(*)
  Product3 : Product  Multiplication=Matrix(*)
  Reshape : Reshape  OutputDimensionality=Column vector (2-D)
  Terminator4 : Terminator
  Terminator5 : Terminator
  f1r : Outport
  wires:
  qdot/1 -> Demux3/1
  q/1 -> Demux2/1
  Demux3/2 -> [q2dot]
  Demux3/1 -> [q1dot]
  Demux2/2 -> [q2]
  Demux2/1 -> [q1]
  r1/1 -> [r1]
  Constant/1 -> Product3/1
  [f1r] -> f1r/1
  [q2dot] -> Terminator4/1
  [q2] -> Terminator5/1
  [q1dot] -> Mux/2
  [q1] -> Mux/1
  Mux/1 -> Reshape/1
  Reshape/1 -> Product3/2
  Constant1/1 -> Product1/1
  [r1] -> Product1/2
  Product3/1 -> Add/1
  Product1/1 -> Add/2
  Add/1 -> [f1r]

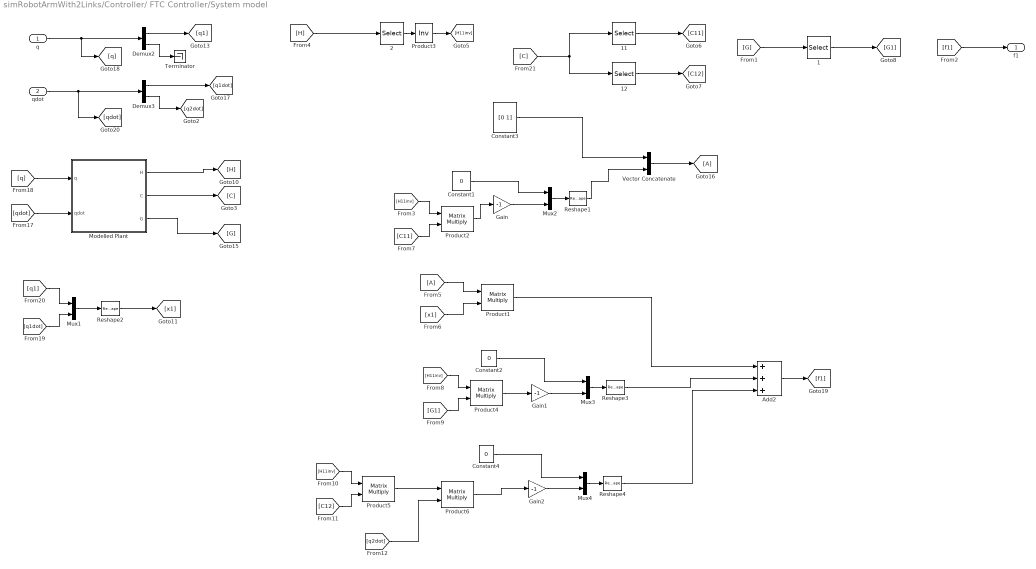
== system simRobotArmWith2Links/Controller/ FTC Controller/System model ==
  q : Inport
  qdot : Inport  Port=2
  1 : Selector  NumberOfDimensions=2  InputPortWidth=3  IndexOptions=Index vector (dialog),Index vector (dialog)  Indices=1,1  OutputSizes=1,1
  11 : Selector  NumberOfDimensions=2  InputPortWidth=3  IndexOptions=Index vector (dialog),Index vector (dialog)  Indices=1,1  OutputSizes=1,1
  12 : Selector  NumberOfDimensions=2  InputPortWidth=3  IndexOptions=Index vector (dialog),Index vector (dialog)  Indices=1,2  OutputSizes=1,1
  2 : Selector  NumberOfDimensions=2  InputPortWidth=3  IndexOptions=Index vector (dialog),Index vector (dialog)  Indices=1,1  OutputSizes=1,1
  Add2 : Sum  Inputs=+++
  Constant1 : Constant  Value=0  VectorParams1D=off
  Constant2 : Constant  Value=0  VectorParams1D=off
  Constant3 : Constant  Value=[0 1]  VectorParams1D=off
  Constant4 : Constant  Value=0  VectorParams1D=off
  Demux2 : Demux  Outputs=2
  Demux3 : Demux  Outputs=2
  Gain : Gain  Gain=-1
  Gain1 : Gain  Gain=-1
  Gain2 : Gain  Gain=-1
  Modelled Plant : Subsystem  TreatAsAtomicUnit=on
  Mux{1..4} (4 alike) : Mux  Inputs=2
  Product{1..2,4..6} (5 alike) : Product  Multiplication=Matrix(*)  RndMeth=Zero
  Product3 : Product  Inputs=/  Multiplication=Matrix(*)  RndMeth=Zero
  Reshape1 : Reshape  OutputDimensionality=Row vector (2-D)
  Reshape2 : Reshape  OutputDimensionality=Column vector (2-D)
  Reshape3 : Reshape  OutputDimensionality=Column vector (2-D)
  Reshape4 : Reshape  OutputDimensionality=Column vector (2-D)
  Terminator : Terminator
  Vector Concatenate : Concatenate  Mode=Multidimensional array
  f1 : Outport
  wires:
  [f1] -> f1/1
  [C] -> 12/1, 11/1
  11/1 -> [C11]
  12/1 -> [C12]
  [G] -> 1/1
  1/1 -> [G1]
  qdot/1 -> [qdot], Demux3/1
  q/1 -> [q], Demux2/1
  Demux3/2 -> [q2dot]
  Demux3/1 -> [q1dot]
  Demux2/2 -> Terminator/1
  Demux2/1 -> [q1]
  [H] -> 2/1
  2/1 -> Product3/1
  Product3/1 -> [H11inv]
  Product1/1 -> Add2/1
  Add2/1 -> [f1]
  [H11inv] -> Product2/1
  [C11] -> Product2/2
  Modelled Plant/1(H) -> [H]
  Modelled Plant/2(C) -> [C]
  Modelled Plant/3(G) -> [G]
  [qdot] -> Modelled Plant/2(qdot)
  [q] -> Modelled Plant/1(q)
  [q1dot] -> Mux1/2
  [q1] -> Mux1/1
  Mux1/1 -> Reshape2/1
  Reshape2/1 -> [x1]
  Product2/1 -> Gain/1
  Constant1/1 -> Mux2/1
  Mux2/1 -> Reshape1/1
  Constant3/1 -> Vector Concatenate/1
  Reshape1/1 -> Vector Concatenate/2
  Vector Concatenate/1 -> [A]
  [A] -> Product1/1
  [x1] -> Product1/2
  [H11inv] -> Product4/1
  [G1] -> Product4/2
  Gain/1 -> Mux2/2
  Product4/1 -> Gain1/1
  Constant2/1 -> Mux3/1
  Mux3/1 -> Reshape3/1
  Gain1/1 -> Mux3/2
  [H11inv] -> Product5/1
  [C12] -> Product5/2
  Constant4/1 -> Mux4/1
  Mux4/1 -> Reshape4/1
  Gain2/1 -> Mux4/2
  Product5/1 -> Product6/1
  [q2dot] -> Product6/2
  Product6/1 -> Gain2/1
  Reshape3/1 -> Add2/2
  Reshape4/1 -> Add2/3

== system simRobotArmWith2Links/Controller/Modelled Plant/get Plant Parameters ==
  H : Inport
  C : Inport  Port=2
  G : Inport  Port=3
  qdot : Inport  Port=4
  {1,5,7,11} (4 alike) : Selector  NumberOfDimensions=2  InputPortWidth=3  IndexOptions=Index vector (dialog),Index vector (dialog)  Indices=1,1  OutputSizes=1,1
  12 : Selector  NumberOfDimensions=2  InputPortWidth=3  IndexOptions=Index vector (dialog),Index vector (dialog)  Indices=1,2  OutputSizes=1,1
  2 : Selector  NumberOfDimensions=2  InputPortWidth=3  IndexOptions=Index vector (dialog),Index vector (dialog)  Indices=1,2  OutputSizes=1,1
  {3,6,8,21} (4 alike) : Selector  NumberOfDimensions=2  InputPortWidth=3  IndexOptions=Index vector (dialog),Index vector (dialog)  Indices=2,1  OutputSizes=1,1
  22 : Selector  NumberOfDimensions=2  InputPortWidth=3  IndexOptions=Index vector (dialog),Index vector (dialog)  Indices=2,2  OutputSizes=1,1
  4 : Selector  NumberOfDimensions=2  InputPortWidth=3  IndexOptions=Index vector (dialog),Index vector (dialog)  Indices=2,2  OutputSizes=1,1
  Bus Creator : BusCreator  Inputs=15
  Product5 : Product  Multiplication=Matrix(*)  RndMeth=Zero
  Sum of Elements1 : Sum
  busData : Outport
  wires:
  2/1 -> Bus Creator/9  "C12"
  21/1 -> Bus Creator/6  "H21"
  22/1 -> Bus Creator/7  "H22"
  4/1 -> Bus Creator/11  "C22"
  6/1 -> Bus Creator/13  "G_2"
  1/1 -> Bus Creator/8  "C11"
  5/1 -> Bus Creator/12  "G_1"
  12/1 -> Bus Creator/5  "H12"
  3/1 -> Bus Creator/10  "C21"
  11/1 -> Bus Creator/4  "H11"
  [H] -> 11/1, 12/1, 21/1, 22/1
  [C] -> 1/1, 2/1, 4/1, 3/1
  [G] -> 6/1, 5/1
  [C] -> Product5/1
  [qdot] -> Product5/2
  Product5/1 -> Sum of Elements1/1
  [G] -> Sum of Elements1/2
  Sum of Elements1/1 -> 7/1, 8/1
  7/1 -> Bus Creator/14  "phi1"
  8/1 -> Bus Creator/15  "phi2"
  [G] -> Bus Creator/3
  Bus Creator/1 -> busData/1
  [C] -> Bus Creator/2
  [H] -> Bus Creator/1
  H/1 -> [H]  "H"
  C/1 -> [C]  "C"
  G/1 -> [G]  "G"
  qdot/1 -> [qdot]

== system simRobotArmWith2Links/Controller/Modelled Plant/getC ==
  s2 : Inport
  q1dot : Inport  Port=2
  q2dot : Inport  Port=3
  C calculation 1 : Subsystem
  C calculation 2 : Subsystem
  Gain2 : Gain  Gain=m2*l1*lc2
  Terminator : Terminator
  C : Outport
  wires:
  s2/1 -> [s2]
  q1dot/1 -> [q1dot]
  q2dot/1 -> [q2dot]
  [s2] -> Gain2/1
  Gain2/1 -> [h]
  [q1dot] -> C calculation 1/1(q1dot)
  [q2dot] -> C calculation 1/2(q2dot)
  [h] -> C calculation 1/3(h)
  [q1dot] -> C calculation 2/1(q1dot)
  [q2dot] -> C calculation 2/2(q2dot)
  [h] -> C calculation 2/3(h)
  [C] -> C/1
  C calculation 2/1(C) -> [C]
  C calculation 1/1(C) -> Terminator/1

== system simRobotArmWith2Links/Controller/Modelled Plant/getG ==
  c1 : Inport
  c12 : Inport  Port=2
  Add : Sum
  Gain : Gain  Gain=(m1*lc1+m2*l1)*g
  Gain1 : Gain  Gain=m2*g*lc2
  Gain2 : Gain
  Gain4 : Gain  Gain=lc2*m2*g
  Matrix Concatenate2 : Concatenate  Mode=Multidimensional array
  G : Outport
  wires:
  [c12] -> Gain4/1
  Gain4/1 -> [G21]
  c12/1 -> [c12]
  c1/1 -> [c1]
  Matrix Concatenate2/1 -> Gain2/1
  [G11] -> Matrix Concatenate2/1
  [G21] -> Matrix Concatenate2/2
  [c1] -> Gain/1
  Gain/1 -> Add/1
  [c12] -> Gain1/1
  Gain1/1 -> Add/2
  Add/1 -> [G11]
  Gain2/1 -> G/1

== system simRobotArmWith2Links/Controller/Modelled Plant/getH ==
  c2 : Inport
  Constant1 : Constant  Value=I1 + I2 + m1*lc1^2 + m2*(l1^2+lc2^2)  VectorParams1D=off
  Constant2 : Constant  Value=I2+m2*lc2^2  VectorParams1D=off
  Constant3 : Constant  Value=I2+m2*lc2^2  VectorParams1D=off
  Gain : Gain  Gain=m2*2*l1*lc2
  Gain1 : Gain  Gain=m2*l1*lc2
  Matrix Concatenate : Concatenate  Mode=Multidimensional array  ConcatenateDimension=2
  Matrix Concatenate1 : Concatenate  Mode=Multidimensional array  ConcatenateDimension=2
  Matrix Concatenate2 : Concatenate  Mode=Multidimensional array
  Sum : Sum
  Sum1 : Sum
  H : Outport
  wires:
  [H11] -> Matrix Concatenate/1
  [H12] -> Matrix Concatenate/2
  Matrix Concatenate/1 -> Matrix Concatenate2/1
  Matrix Concatenate1/1 -> Matrix Concatenate2/2
  [H21] -> Matrix Concatenate1/1
  [H22] -> Matrix Concatenate1/2
  Matrix Concatenate2/1 -> H/1
  c2/1 -> [c2]
  [c2] -> Gain/1
  Gain/1 -> Sum/1
  Constant1/1 -> Sum/2
  Sum/1 -> [H11]
  [c2] -> Gain1/1
  Gain1/1 -> Sum1/1
  Constant2/1 -> Sum1/2
  Sum1/1 -> [H12], [H21]
  Constant3/1 -> [H22]

== system simRobotArmWith2Links/Controller/Partial FBL q2 Controller/Collocated q2 Controller ==
  r : Inport
  rdot : Inport  Port=2
  q : Inport  Port=3
  qdot : Inport  Port=4
  Add3 : Sum
  Gain2 : Gain  Gain=-K1
  Gain3 : Gain  Gain=-K2
  sum1 : Sum  Inputs=+-
  sum2 : Sum  Inputs=+-
  v : Outport
  wires:
  Add3/1 -> [v]
  Gain3/1 -> Add3/2
  Gain2/1 -> Add3/1
  [e] -> Gain3/1
  [edot] -> Gain2/1
  qdot/1 -> [qdot]  "qdot"
  q/1 -> [q]  "q"
  [q] -> sum1/1
  [r] -> sum1/2
  sum1/1 -> [e]  "e"
  r/1 -> [r]  "r"
  [v] -> v/1  "v"
  [qdot] -> sum2/1
  [rdot] -> sum2/2
  sum2/1 -> [edot]  "edot"
  rdot/1 -> [rdot]  "rdot"

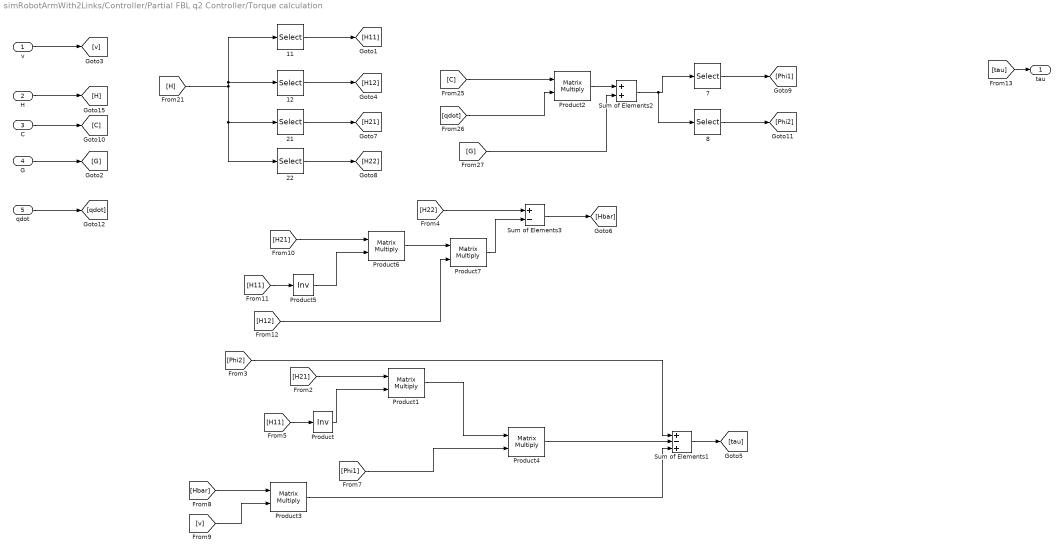
== system simRobotArmWith2Links/Controller/Partial FBL q2 Controller/Torque calculation ==
  v : Inport
  H : Inport  Port=2
  C : Inport  Port=3
  G : Inport  Port=4
  qdot : Inport  Port=5
  11 : Selector  NumberOfDimensions=2  InputPortWidth=3  IndexOptions=Index vector (dialog),Index vector (dialog)  Indices=1,1  OutputSizes=1,1
  12 : Selector  NumberOfDimensions=2  InputPortWidth=3  IndexOptions=Index vector (dialog),Index vector (dialog)  Indices=1,2  OutputSizes=1,1
  21 : Selector  NumberOfDimensions=2  InputPortWidth=3  IndexOptions=Index vector (dialog),Index vector (dialog)  Indices=2,1  OutputSizes=1,1
  22 : Selector  NumberOfDimensions=2  InputPortWidth=3  IndexOptions=Index vector (dialog),Index vector (dialog)  Indices=2,2  OutputSizes=1,1
  7 : Selector  NumberOfDimensions=2  InputPortWidth=3  IndexOptions=Index vector (dialog),Index vector (dialog)  Indices=1,1  OutputSizes=1,1
  8 : Selector  NumberOfDimensions=2  InputPortWidth=3  IndexOptions=Index vector (dialog),Index vector (dialog)  Indices=2,1  OutputSizes=1,1
  Product : Product  Inputs=/  Multiplication=Matrix(*)  RndMeth=Zero
  Product{1..4,6..7} (6 alike) : Product  Multiplication=Matrix(*)  RndMeth=Zero
  Product5 : Product  Inputs=/  Multiplication=Matrix(*)  RndMeth=Zero
  Sum of Elements1 : Sum  Inputs=+-+
  Sum of Elements2 : Sum
  Sum of Elements3 : Sum  Inputs=+-
  tau : Outport
  wires:
  [tau] -> tau/1
  v/1 -> [v]
  [H11] -> Product/1
  [H21] -> Product1/1
  Product/1 -> Product1/2
  Product1/1 -> Product4/1
  [Hbar] -> Product3/1
  [v] -> Product3/2
  Sum of Elements1/1 -> [tau]
  [H11] -> Product5/1
  [H21] -> Product6/1
  Product5/1 -> Product6/2
  Product6/1 -> Product7/1
  [H12] -> Product7/2
  [H22] -> Sum of Elements3/1
  Product7/1 -> Sum of Elements3/2
  Sum of Elements3/1 -> [Hbar]
  [Phi1] -> Product4/2
  [Phi2] -> Sum of Elements1/1
  Product4/1 -> Sum of Elements1/2
  Product3/1 -> Sum of Elements1/3
  C/1 -> [C]
  H/1 -> [H]
  G/1 -> [G]
  [H] -> 11/1, 12/1, 21/1, 22/1
  [C] -> Product2/1
  [qdot] -> Product2/2
  Product2/1 -> Sum of Elements2/1
  [G] -> Sum of Elements2/2
  Sum of Elements2/1 -> 7/1, 8/1
  11/1 -> [H11]
  12/1 -> [H12]
  21/1 -> [H21]
  22/1 -> [H22]
  7/1 -> [Phi1]
  8/1 -> [Phi2]
  qdot/1 -> [qdot]

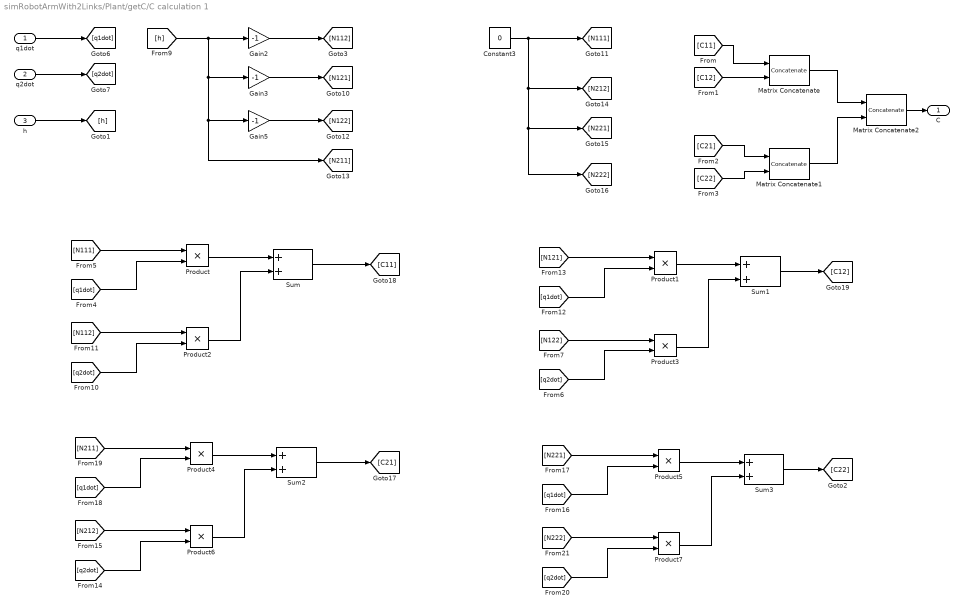
== system simRobotArmWith2Links/Plant/getC/C calculation 1 ==
  q1dot : Inport
  q2dot : Inport  Port=2
  h : Inport  Port=3
  Constant3 : Constant  Value=0  VectorParams1D=off
  Gain2 : Gain  Gain=-1
  Gain3 : Gain  Gain=-1
  Gain5 : Gain  Gain=-1
  Matrix Concatenate : Concatenate  Mode=Multidimensional array  ConcatenateDimension=2
  Matrix Concatenate1 : Concatenate  Mode=Multidimensional array  ConcatenateDimension=2
  Matrix Concatenate2 : Concatenate  Mode=Multidimensional array
  Product{,1..7} (8 alike) : Product  RndMeth=Zero
  Sum{,1..3} (4 alike) : Sum
  C : Outport
  wires:
  q2dot/1 -> [q2dot]
  q1dot/1 -> [q1dot]
  [N111] -> Product/1
  Product/1 -> Sum/1
  [q1dot] -> Product/2
  [N112] -> Product2/1
  Product2/1 -> Sum/2
  [q2dot] -> Product2/2
  Sum/1 -> [C11]
  [N121] -> Product1/1
  Product1/1 -> Sum1/1
  [q1dot] -> Product1/2
  [N122] -> Product3/1
  Product3/1 -> Sum1/2
  [q2dot] -> Product3/2
  Sum1/1 -> [C12]
  [N211] -> Product4/1
  Product4/1 -> Sum2/1
  [q1dot] -> Product4/2
  [N212] -> Product6/1
  Product6/1 -> Sum2/2
  [q2dot] -> Product6/2
  Sum2/1 -> [C21]
  [N221] -> Product5/1
  Product5/1 -> Sum3/1
  [q1dot] -> Product5/2
  [N222] -> Product7/1
  Product7/1 -> Sum3/2
  [q2dot] -> Product7/2
  Constant3/1 -> [N111], [N212], [N221], [N222]
  [h] -> Gain2/1, Gain3/1, Gain5/1, [N211]
  Gain2/1 -> [N112]
  Gain3/1 -> [N121]
  Gain5/1 -> [N122]
  h/1 -> [h]
  Sum3/1 -> [C22]
  Matrix Concatenate2/1 -> C/1
  [C22] -> Matrix Concatenate1/2
  [C21] -> Matrix Concatenate1/1
  Matrix Concatenate1/1 -> Matrix Concatenate2/2
  Matrix Concatenate/1 -> Matrix Concatenate2/1
  [C12] -> Matrix Concatenate/2
  [C11] -> Matrix Concatenate/1

== system simRobotArmWith2Links/Plant/getC/C calculation 2 ==
  q1dot : Inport
  q2dot : Inport  Port=2
  h : Inport  Port=3
  Constant1 : Constant  Value=0  VectorParams1D=off
  Gain6 : Gain  Gain=-2
  Gain7 : Gain  Gain=-1
  Matrix Concatenate : Concatenate  Mode=Multidimensional array  ConcatenateDimension=2
  Matrix Concatenate1 : Concatenate  Mode=Multidimensional array  ConcatenateDimension=2
  Matrix Concatenate2 : Concatenate  Mode=Multidimensional array
  Product10 : Product  RndMeth=Zero
  Product8 : Product  RndMeth=Zero
  Product9 : Product  RndMeth=Zero
  C : Outport
  wires:
  h/1 -> [h]
  q1dot/1 -> [q1dot]
  q2dot/1 -> [q2dot]
  [h] -> Gain6/1
  [h] -> Gain7/1
  Gain7/1 -> Product10/2
  Product10/1 -> [C12]
  Constant1/1 -> [C22]
  [h] -> Product8/2
  [q1dot] -> Product8/1
  Product8/1 -> [C21]
  Gain6/1 -> Product9/2
  Product9/1 -> [C11]
  [q2dot] -> Product9/1
  Matrix Concatenate2/1 -> C/1
  [C22] -> Matrix Concatenate1/2
  [C21] -> Matrix Concatenate1/1
  Matrix Concatenate1/1 -> Matrix Concatenate2/2
  Matrix Concatenate/1 -> Matrix Concatenate2/1
  [C12] -> Matrix Concatenate/2
  [C11] -> Matrix Concatenate/1
  [q2dot] -> Product10/1

== system simRobotArmWith2Links/Controller/ FTC Controller/System model/Modelled Plant ==
  q : Inport
  qdot : Inport  Port=2
  Demux : Demux  Outputs=2
  Demux1 : Demux  Outputs=2
  Demux2 : Demux  Outputs=2
  Sum of Elements : Sum  Inputs=+
  Terminator4 : Terminator
  Terminator5 : Terminator
  Terminator6 : Terminator
  Trigonometric Function : Trigonometry
  Trigonometric Function1 : Trigonometry  Operator=cos
  Trigonometric Function2 : Trigonometry
  Trigonometric Function3 : Trigonometry  Operator=cos
  get Plant Parameters : Subsystem
  getC : Subsystem
  getG : Subsystem
  getH : Subsystem
  H : Outport
  C : Outport  Port=2
  G : Outport  Port=3
  wires:
  [c2] -> getH/1(c2)
  [s2] -> getC/1(s2)
  [q1dot] -> getC/2(q1dot)
  [q2dot] -> getC/3(q2dot)
  getH/1(H) -> [H]
  getC/1(C) -> [C]
  [c1] -> getG/1(c1)
  [c12] -> getG/2(c12)
  getG/1(G) -> [G]
  q/1 -> Trigonometric Function/1, Trigonometric Function1/1, Sum of Elements/1
  Trigonometric Function/1 -> Demux/1
  Demux/1 -> Terminator4/1
  Demux/2 -> [s2]
  Demux1/1 -> [c1]
  Demux1/2 -> [c2]
  Trigonometric Function1/1 -> Demux1/1
  Sum of Elements/1 -> Trigonometric Function2/1, Trigonometric Function3/1
  Trigonometric Function2/1 -> Terminator5/1
  qdot/1 -> Demux2/1, [qdot]
  Demux2/1 -> [q1dot]
  Demux2/2 -> [q2dot]
  Trigonometric Function3/1 -> [c12]
  [H] -> H/1
  [C] -> C/1
  [G] -> G/1
  get Plant Parameters/1(busData) -> Terminator6/1  "ModeledSystem"
  [C] -> get Plant Parameters/2(C)
  [H] -> get Plant Parameters/1(H)
  [G] -> get Plant Parameters/3(G)
  [qdot] -> get Plant Parameters/4(qdot)

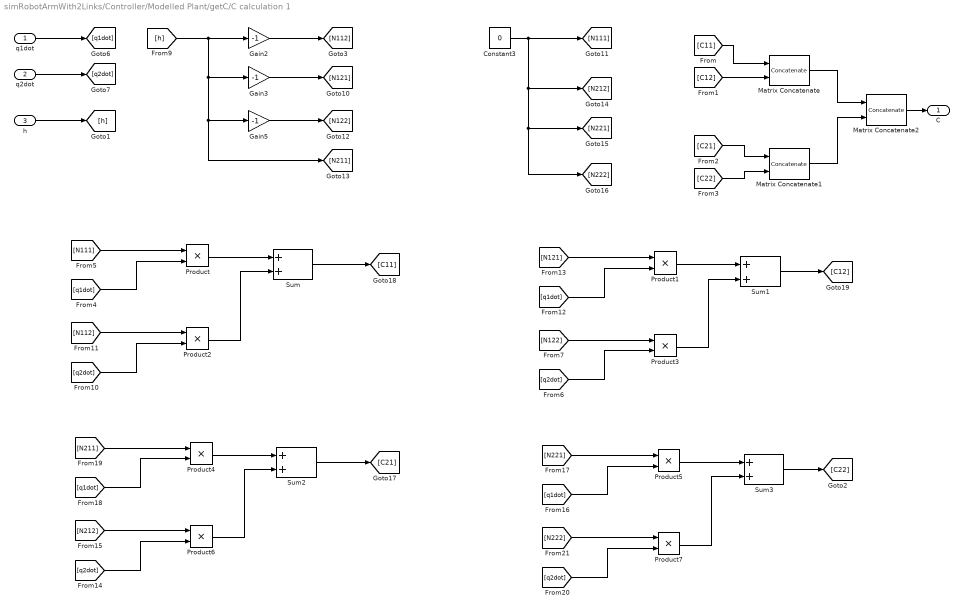
== system simRobotArmWith2Links/Controller/Modelled Plant/getC/C calculation 1 ==
  q1dot : Inport
  q2dot : Inport  Port=2
  h : Inport  Port=3
  Constant3 : Constant  Value=0  VectorParams1D=off
  Gain2 : Gain  Gain=-1
  Gain3 : Gain  Gain=-1
  Gain5 : Gain  Gain=-1
  Matrix Concatenate : Concatenate  Mode=Multidimensional array  ConcatenateDimension=2
  Matrix Concatenate1 : Concatenate  Mode=Multidimensional array  ConcatenateDimension=2
  Matrix Concatenate2 : Concatenate  Mode=Multidimensional array
  Product{,1..7} (8 alike) : Product  RndMeth=Zero
  Sum{,1..3} (4 alike) : Sum
  C : Outport
  wires:
  q2dot/1 -> [q2dot]
  q1dot/1 -> [q1dot]
  [N111] -> Product/1
  Product/1 -> Sum/1
  [q1dot] -> Product/2
  [N112] -> Product2/1
  Product2/1 -> Sum/2
  [q2dot] -> Product2/2
  Sum/1 -> [C11]
  [N121] -> Product1/1
  Product1/1 -> Sum1/1
  [q1dot] -> Product1/2
  [N122] -> Product3/1
  Product3/1 -> Sum1/2
  [q2dot] -> Product3/2
  Sum1/1 -> [C12]
  [N211] -> Product4/1
  Product4/1 -> Sum2/1
  [q1dot] -> Product4/2
  [N212] -> Product6/1
  Product6/1 -> Sum2/2
  [q2dot] -> Product6/2
  Sum2/1 -> [C21]
  [N221] -> Product5/1
  Product5/1 -> Sum3/1
  [q1dot] -> Product5/2
  [N222] -> Product7/1
  Product7/1 -> Sum3/2
  [q2dot] -> Product7/2
  Constant3/1 -> [N111], [N212], [N221], [N222]
  [h] -> Gain2/1, Gain3/1, Gain5/1, [N211]
  Gain2/1 -> [N112]
  Gain3/1 -> [N121]
  Gain5/1 -> [N122]
  h/1 -> [h]
  Sum3/1 -> [C22]
  Matrix Concatenate2/1 -> C/1
  [C22] -> Matrix Concatenate1/2
  [C21] -> Matrix Concatenate1/1
  Matrix Concatenate1/1 -> Matrix Concatenate2/2
  Matrix Concatenate/1 -> Matrix Concatenate2/1
  [C12] -> Matrix Concatenate/2
  [C11] -> Matrix Concatenate/1

== system simRobotArmWith2Links/Controller/Modelled Plant/getC/C calculation 2 ==
  q1dot : Inport
  q2dot : Inport  Port=2
  h : Inport  Port=3
  Constant1 : Constant  Value=0  VectorParams1D=off
  Gain6 : Gain  Gain=-2
  Gain7 : Gain  Gain=-1
  Matrix Concatenate : Concatenate  Mode=Multidimensional array  ConcatenateDimension=2
  Matrix Concatenate1 : Concatenate  Mode=Multidimensional array  ConcatenateDimension=2
  Matrix Concatenate2 : Concatenate  Mode=Multidimensional array
  Product10 : Product  RndMeth=Zero
  Product8 : Product  RndMeth=Zero
  Product9 : Product  RndMeth=Zero
  C : Outport
  wires:
  h/1 -> [h]
  q1dot/1 -> [q1dot]
  q2dot/1 -> [q2dot]
  [h] -> Gain6/1
  [h] -> Gain7/1
  Gain7/1 -> Product10/2
  Product10/1 -> [C12]
  Constant1/1 -> [C22]
  [h] -> Product8/2
  [q1dot] -> Product8/1
  Product8/1 -> [C21]
  Gain6/1 -> Product9/2
  Product9/1 -> [C11]
  [q2dot] -> Product9/1
  Matrix Concatenate2/1 -> C/1
  [C22] -> Matrix Concatenate1/2
  [C21] -> Matrix Concatenate1/1
  Matrix Concatenate1/1 -> Matrix Concatenate2/2
  Matrix Concatenate/1 -> Matrix Concatenate2/1
  [C12] -> Matrix Concatenate/2
  [C11] -> Matrix Concatenate/1
  [q2dot] -> Product10/1
